simulink model "ddcfilterchaindemo_cosim"  (Simulink 8.3)
settings: Solver=FixedStepDiscrete  SolverMode=SingleTasking  StartTime=0.0  StopTime=20000  FixedStep=1  RelTol=1e-3
PreLoadFcn:
  | x=[ zeros(1,5), chirp(0:1999,0,1999,0.4)];
  | x_in=fi(x,1,20,18);
undefined symbols (not defined in the file or in its folder): clk, filter
libraries: dspmlti4 x3, dspmisc x1, dspsrcs4 x1, modelsimlib x1
settings Model: Creator=The MathWorks Inc.
settings OptimizationCC: ExpressionDepthLimit=2147483647  InitFltsAndDblsToZero=on  BufferReusableBoundary=off
settings DebuggingCC: SaveWithParameterizedLinksMsg=none  CheckExecutionContextPreStartOutputMsg=on  CheckExecutionContextRuntimeOutputMsg=on  SignalResolutionControl=TryResolveAllWithWarning  MultiTaskDSMMsg=warning  MultiTaskCondExecSysMsg=none  IntegerOverflowMsg=none  FcnCallInpInsideContextMsg=UseLocalSettings  BusObjectLabelMismatch=none  StrictBusMsg=None
settings RTWCC: IncludeERTFirstTime=on
settings GRTTargetCC: TargetFcnLib=ansi_tfl_tmw.mat

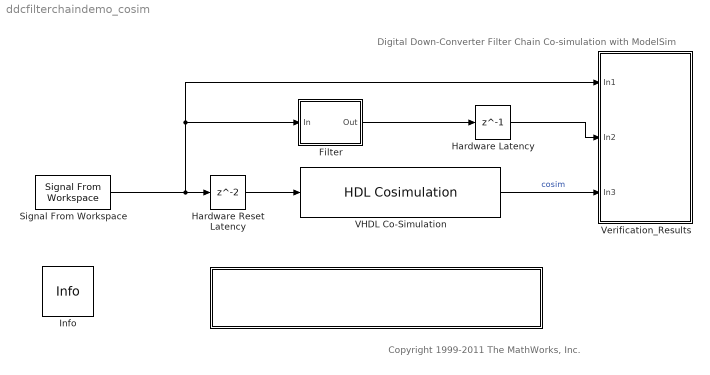
== system ddcfilterchaindemo_cosim ==
  note: Digital Down-Converter Filter Chain
      | Co-simulation with ModelSim
  note: Copyright 1999-2011 The MathWorks, Inc.
  " " : Subsystem  mask(VHDL DDC Filter Chain Demo Info){}
      settings: OpenFcn=vsim('tclstart',ddcdemolinkcmds,'socketsimulink',4449)
      mask Display: disp(['vsim(''tclstart'',ddcdemolinkcmds,''socketsimulink'',4449)', char(10),'%', 'Double click to launch a new ModelSim'])
  Filter : Subsystem  Tag=BlockMethodSubSystem
  Hardware Latency : Delay  DelayLength=1  InputProcessing=Inherited
  Hardware Reset Latency : Delay  InputProcessing=Inherited
  Info : dspmisc/Info  SystemSampleTime=-1
  Signal From Workspace : dspsrcs4/Signal From Workspace  X=x_in  Ts=10  nsamps=1  OutputAfterFinalValue=Setting to zero  ignoreOrWarnInputAndFrameLengths=off
  VHDL Co-Simulation : modelsimlib/HDL Cosimulation  PortPaths=/filter/filter_in;/filter/filter_out  PortModes=[1 2 ]  PortTimes=[-1,2560]  PortSigns=[-1 -1 ]  PortFracLengths=[0,0]  CommLocal=on  CommSharedMemory=off  CommPortNumber=4449  CommShowInfo=off  ClockPaths=filter/clk  ClockModes=[2 ]  ClockTimes=[10]  TclPreSimCommand="force sim:/filter/clk_enable 1; force sim:/filter/reset 1 0 ns, 0 {22 ns}; echo \"Running Simulink Cosimulation block.\"; echo [clock format [clock seconds]]"  TclPostSimCommand=force sim:/filter/reset 1  TimingMode=Tick  TimingScaleFactor=1  idxCellArray={'UNUSED_VAR'}  CosimBypass=Full Simulation  AllowDirectFeedthrough=off  ProductName=EDA Simulator Link MQ  RunAutoTimescale=off  HdlClocks=0  PreRunTime=0  PreRunTimeUnit=ns
  Verification_Results : Subsystem
      mask Display:
      | port_label('input',1,'Input');
      | port_label('input',2,'Sim');
      | port_label('input',3,'HDL Co-Sim');
  wires:
  Signal From Workspace/1 -> Hardware Reset Latency/1, Verification_Results/1(In1), Filter/1(In)
  VHDL Co-Simulation/1 -> Verification_Results/3(In3)  "cosim"
  Hardware Reset Latency/1 -> VHDL Co-Simulation/1
  Hardware Latency/1 -> Verification_Results/2(In2)
  Filter/1(Out) -> Hardware Latency/1

== system ddcfilterchaindemo_cosim/  ==

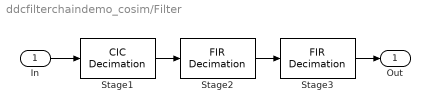
== system ddcfilterchaindemo_cosim/Filter ==
  In : Inport
  Stage1 : dspmlti4/CIC Decimation  Tag=BlockMethodSubSystem  filtFrom=Dialog  filtobj=Hm_decim  ftype=Decimator  R=64  M=1  N=5  filterInternals=Full precision  BPS=[49 43 37 33 28 26 25 24 23 23]  FLPS=0  outputWordLength=20  outputFracLength=0  launchFVT=off  framing=Maintain input frame rate  RateOptions=Allow multirate processing
  Stage2 : dspmlti4/FIR Decimation  Tag=BlockMethodSubSystem  h=[-0.0008392333984375 -0.001220703125 0.0037384033203125 0.012481689453125 0.0074462890625 -0.026031494140625 -0.0601959228515625 -0.02587890625 0.113571166992188 0.290786743164063 0.372772216796875 0.290786743164063 0.113571166992188 -0.02587890625 -0.0601959228515625 -0.026031494140625 0.0074462890625 0.012481689453125 0.0037384033203125 -0.001220703125 -0.0008392333984375]  D=2  filtStruct=Direct form  framing=Allow multirate processing  inputOffset=0  outputBufInitCond=0  firstCoeffMode=Binary point scaling  firstCoeffWordLength=16  firstCoeffFracLength=16  firstCoeffDataTypeStr=fixdt(1,16,16)  firstCoeffLastDataTypeStr=fixdt(1,16,16)  firstCoeffMin=[]  firstCoeffMax=[]  outputMode=Binary point scaling  outputWordLength=37  outputFracLength=4  outputDataTypeStr=fixdt(1,37,4)  outputLastDataTypeStr=fixdt(1,37,4)  outputMin=[]  outputMax=[]  accumMode=Binary point scaling  accumWordLength=37  accumFracLength=4  accumDataTypeStr=fixdt(1,37,4)  accumLastDataTypeStr=fixdt(1,37,4)  prodOutputMode=Binary point scaling  prodOutputWordLength=35  prodOutputFracLength=4  prodOutputDataTypeStr=fixdt(1,35,4)  prodOutputLastDataTypeStr=fixdt(1,35,4)  roundingMode=Nearest  overflowMode=off  FilterSource=Specify via dialog  FilterObject=Hm_firdecim
  Stage3 : dspmlti4/FIR Decimation  Tag=BlockMethodSubSystem  h=[0.004058837890625 -0.0002288818359375 -0.0023345947265625 -0.0028839111328125 -0.0003814697265625 0.0033416748046875 0.0042266845703125 0.0003662109375 -0.0050811767578125 -0.0062255859375 -0.0005340576171875 0.0072174072265625 0.0086517333984375 0.00048828125 -0.0103302001953125 -0.0121612548828125 -0.000640869140625 0.0144500732421875 0.0168609619140625 0.0005950927734375 -0.020782470703125 -0.024261474609375 -0.0007171630859375 0.0310821533203125 0.0370330810546875 0.0006561279296875 -0.05291748046875 -0.067779541015625 -0.0007476806640625 0.13665771484375 0.275588989257813 0.333999633789063 0.275588989257813 0.13665771484375 -0.0007476806640625 -0.067779541015625 -0.05291748046875 0.0006561279296875 0.0370330810546875 0.0310821533203125 -0.0007171630859375 -0.024261474609375 -0.020782470703125 0.0005950927734375 0.0168609619140625 0.0144500732421875 -0.000640869140625 -0.0121612548828125 -0.0103302001953125 0.00048828125 0.0086517333984375 0.0072174072265625 -0.0005340576171875 -0.0062255859375 -0.0050811767578125 0.0003662109375 0.0042266845703125 0.0033416748046875 -0.0003814697265625 -0.0028839111328125 -0.0023345947265625 -0.0002288818359375 0.004058837890625]  D=2  filtStruct=Direct form  framing=Allow multirate processing  inputOffset=0  outputBufInitCond=0  firstCoeffMode=Binary point scaling  firstCoeffWordLength=16  firstCoeffFracLength=16  firstCoeffDataTypeStr=fixdt(1,16,16)  firstCoeffLastDataTypeStr=fixdt(1,16,16)  firstCoeffMin=[]  firstCoeffMax=[]  outputMode=Binary point scaling  outputWordLength=20  outputFracLength=-12  outputDataTypeStr=fixdt(1,20,-12)  outputLastDataTypeStr=fixdt(1,20,-12)  outputMin=[]  outputMax=[]  accumMode=Binary point scaling  accumWordLength=37  accumFracLength=4  accumDataTypeStr=fixdt(1,37,4)  accumLastDataTypeStr=fixdt(1,37,4)  prodOutputMode=Binary point scaling  prodOutputWordLength=35  prodOutputFracLength=4  prodOutputDataTypeStr=fixdt(1,35,4)  prodOutputLastDataTypeStr=fixdt(1,35,4)  roundingMode=Nearest  overflowMode=on  FilterSource=Specify via dialog  FilterObject=Hm_firdecim
  Out : Outport
  wires:
  In/1 -> Stage1/1
  Stage1/1 -> Stage2/1
  Stage2/1 -> Stage3/1
  Stage3/1 -> Out/1

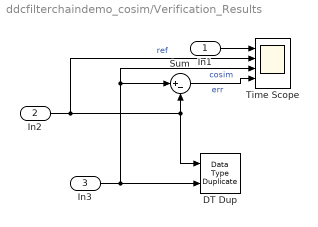
== system ddcfilterchaindemo_cosim/Verification_Results ==
  In1 : Inport
  In2 : Inport  Port=2
  In3 : Inport  Port=3
  DT Dup : DataTypeDuplicate
  Sum : Sum  Inputs=|+-
  Time Scope : Scope  NumInputPorts=4
      settings: TimeRange=20000  YMin=-1~-500000~-500000~-1  YMax=1~1e+006~1e+006~1  DataFormat=Structure
  wires:
  In3/1 -> DT Dup/2, Sum/1, Time Scope/3  "cosim"
  Sum/1 -> Time Scope/4  "err"
  In2/1 -> DT Dup/1, Sum/2, Time Scope/2  "ref"
  In1/1 -> Time Scope/1
